simulink model "Sfun_test"  (Simulink 8.7)
settings: Solver=ode45  StartTime=0.0  StopTime=1  MaxStep=1e-6  MinStep=1e-7  RelTol=1e-3
settings Model: Creator=wangbingo  LastModifiedBy=wang_bingo
settings DataIOCC: LimitDataPoints=off  SaveFormat=Dataset
settings DebuggingCC: UnderspecifiedInitializationDetection=Simplified  MergeDetectMultiDrivingBlocksExec=error
settings HardwareCC: ProdBitPerPointer=64  ProdLargestAtomicFloat=Float  ProdIntDivRoundTo=Zero  ProdEndianess=LittleEndian  ProdWordSize=64  ProdHWDeviceType=Intel->x86-64 (Windows64)
settings ModelReferenceCC: PropagateSignalLabelsOutOfModel=on
settings ConfigComp: CovModelRefEnable=off

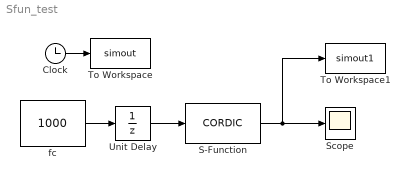
== system Sfun_test ==
  Clock : Clock
  S-Function : S-Function  FunctionName=CORDIC  SFunctionDeploymentMode=off  EnableBusSupport=off
  Scope : Scope
  To Workspace : ToWorkspace  VariableName=simout  SaveFormat=Timeseries  SampleTime=-1
  To Workspace1 : ToWorkspace  VariableName=simout1  SaveFormat=Timeseries  SampleTime=-1
  Unit Delay : UnitDelay  SampleTime=1/750000
  fc : Constant  Value=1000
  wires:
  S-Function/1 -> To Workspace1/1, Scope/1
  fc/1 -> Unit Delay/1
  Unit Delay/1 -> S-Function/1
  Clock/1 -> To Workspace/1
